simulink model "force_ds_test"  (R2020b)
settings: Solver=FixedStepAuto  StartTime=0.0  StopTime=0.4  FixedStep=0.0001  RelTol=1e-3
settings Model: Creator=kika  LastModifiedBy=kika

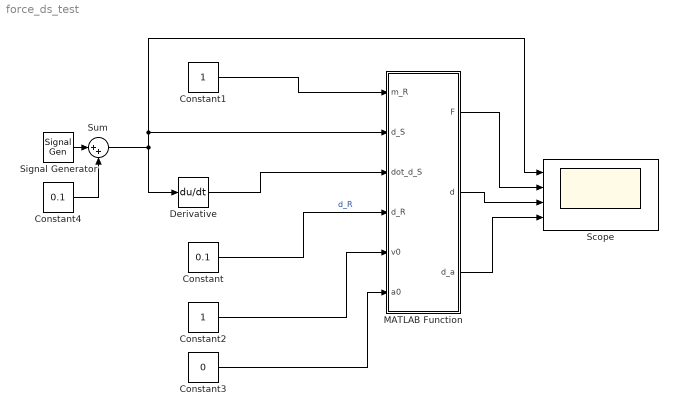
== system force_ds_test ==
  Constant : Constant  Value=0.1
  Constant1 : Constant
  Constant2 : Constant
  Constant3 : Constant  Value=0
  Constant4 : Constant  Value=0.1
  Derivative : Derivative
  MATLAB Function : MATLAB Function  TreatAsAtomicUnit=on
  Scope : Scope  NumInputPorts=4
  Signal Generator : SignalGenerator  Amplitude=0.1  Frequency=100  Units=rad/sec
  Sum : Sum  Inputs=|++
  wires:
  Constant/1 -> MATLAB Function/4(d_R)  "d_R"
  Constant1/1 -> MATLAB Function/1(m_R)
  Constant2/1 -> MATLAB Function/5(v0)
  Constant3/1 -> MATLAB Function/6(a0)
  MATLAB Function/1(F) -> Scope/2
  MATLAB Function/2(d) -> Scope/3
  MATLAB Function/3(d_a) -> Scope/4
  Signal Generator/1 -> Sum/1
  Constant4/1 -> Sum/2
  Sum/1 -> MATLAB Function/2(d_S), Scope/1, Derivative/1
  Derivative/1 -> MATLAB Function/3(dot_d_S)

== matlab function force_ds_test/MATLAB Function ==
  data: m_R input; d_S input; dot_d_S input; F output; d output; d_R input; d_a output; v0 input; a0 input
function [F, d, d_a]= fcn(m_R, d_S, dot_d_S, d_R, v0, a0)


    a_max = 1;
    j_max = 100;
    
    t_da = v0 / a_max;
   
    t_a = a_max / j_max;
    d_a = v0 * t_a + 0.5 * a0 * t_a^2 + 0.1667 * j_max * t_a^2;
   
    
    d = d_R - d_S;

    F = 0;
    
    if d_S < d_R
        if dot_d_S < 0
            F = m_R * sign(v0);
            if d <= d_a
                F = F * d;
            elseif d <= (d_R - d_a)
                F = F * a_max;
            else
                F = F * (d_R - d);
            end
        end
    end
